simulink model "thermostat"  (Simulink 7.8)
settings: Solver=ode45  StartTime=0.0  StopTime=10.0  RelTol=1e-3
settings Model: Creator=rpichard  LastModifiedBy=rpichard
settings OptimizationCC: BlockReduction=off  BooleanDataType=off
settings DebuggingCC: SaveWithParameterizedLinksMsg=none  SignalResolutionControl=TryResolveAllWithWarning  SolverPrmCheckMsg=none  MultiTaskDSMMsg=warning  MultiTaskCondExecSysMsg=none  StrictBusMsg=None
settings HardwareCC: TargetUnknown=on
settings RTWCC: IncludeERTFirstTime=on

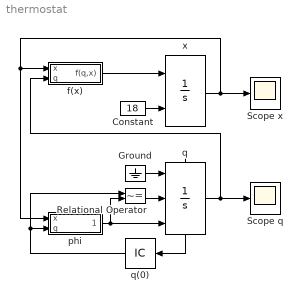
== system thermostat ==
  Constant : Constant  Value=18
  Ground : Ground
  Relational Operator : RelationalOperator  Operator=~=  InputSameDT=on
  Scope q : Scope
      settings: TimeRange=10  YMin=0  YMax=3
  Scope x : Scope
      settings: TimeRange=10  YMin=60  YMax=80
  f(x) : Subsystem  Description=f(x)
  phi : Subsystem  Description=f(x)
  q : Integrator  ExternalReset=rising  InitialConditionSource=external  ShowStatePort=on
  q(0) : InitialCondition
  x : Integrator  InitialConditionSource=external
  wires:
  Constant/1 -> x/2
  f(x)/1(f(q,x)) -> x/1
  x/1 -> Scope x/1, phi/1(x), f(x)/1(x)
  q/1 -> Scope q/1, f(x)/2(q)
  Ground/1 -> q/1
  Relational Operator/1 -> q/2
  phi/1(phi(q,x)) -> q/3, Relational Operator/2
  q(0)/1 -> phi/2(q), Relational Operator/1
  q/State -> q(0)/1

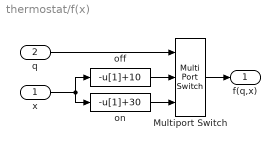
== system thermostat/f(x) ==
  x : Inport
  q : Inport  Port=2
  Multiport Switch : MultiPortSwitch  Inputs=2  zeroidx=off  SaturateOnIntegerOverflow=on  InputSameDT=on
  off : Fcn  Expr=-u[1]+10
  on : Fcn  Expr=-u[1]+30
  f(q,x) : Outport
  wires:
  Multiport Switch/1 -> f(q,x)/1
  off/1 -> Multiport Switch/2
  on/1 -> Multiport Switch/3
  x/1 -> off/1, on/1
  q/1 -> Multiport Switch/1

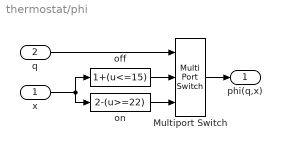
== system thermostat/phi ==
  x : Inport
  q : Inport  Port=2
  Multiport Switch : MultiPortSwitch  Inputs=2  zeroidx=off  SaturateOnIntegerOverflow=on  InputSameDT=on
  off : Fcn  Expr=1+(u<=15)
  on : Fcn  Expr=2-(u>=22)
  phi(q,x) : Outport
  wires:
  x/1 -> on/1, off/1
  on/1 -> Multiport Switch/3
  off/1 -> Multiport Switch/2
  Multiport Switch/1 -> phi(q,x)/1
  q/1 -> Multiport Switch/1
